simulink model "final_heart_sym3_3_Level_fixed"  (R2021a)
settings: Solver=FixedStepDiscrete  StartTime=0.0  StopTime=8  RelTol=1e-3
undefined symbols (not defined in the file): lambda2
(part 1 of 2)
settings Model: DataTypeOverride=Off  FPTShortcutValueString='{{},{''BaselineRun'',1,1,1,''BaselineRun'','''',{},''M'','''',''''}}'  Creator=Ruth Matienzo  LastModifiedBy=Acer
settings OptimizationCC: BlockReduction=off  ConditionallyExecuteInputs=off  DefaultParameterBehavior=Inlined
settings DebuggingCC: SignalRangeChecking=warning  AlgebraicLoopMsg=error  SingleTaskRateTransMsg=error
settings HardwareCC: ProdBitPerPointer=32  ProdBitPerSizeT=32  ProdBitPerPtrDiffT=32  ProdLargestAtomicFloat=None  ProdIntDivRoundTo=Undefined  ProdEndianess=Unspecified  ProdWordSize=32  ProdHWDeviceType=ASIC/FPGA->ASIC/FPGA  TargetBitPerPointer=64  TargetBitPerSizeT=64  TargetBitPerPtrDiffT=64  TargetLongLongMode=on  TargetIntDivRoundTo=Zero  TargetEndianess=LittleEndian  TargetWordSize=64  TargetHWDeviceType=Custom Processor->MATLAB Host Computer  ProdEqTarget=off

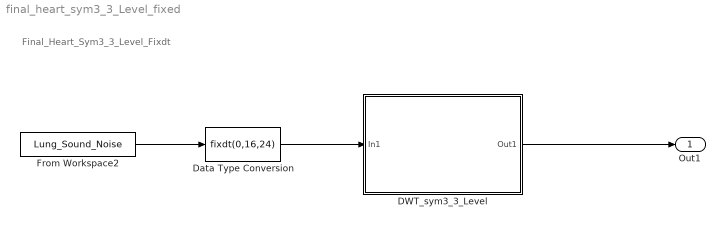
== system final_heart_sym3_3_Level_fixed ==
  note: Final_Heart_Sym3_3_Level_Fixdt
  DWT_sym3_3_Level : Subsystem
  Data Type Conversion : DataTypeConversion  OutDataTypeStr=fixdt(0,16,24)
  From Workspace2 : FromWorkspace  VariableName=Lung_Sound_Noise  OutDataTypeStr=double  SampleTime=1/44100
  Out1 : Outport  OutDataTypeStr=fixdt(1,16,23)  SampleTime=1/44100
  wires:
  Data Type Conversion/1 -> DWT_sym3_3_Level/1(In1)
  DWT_sym3_3_Level/1(Out1) -> Out1/1
  From Workspace2/1 -> Data Type Conversion/1

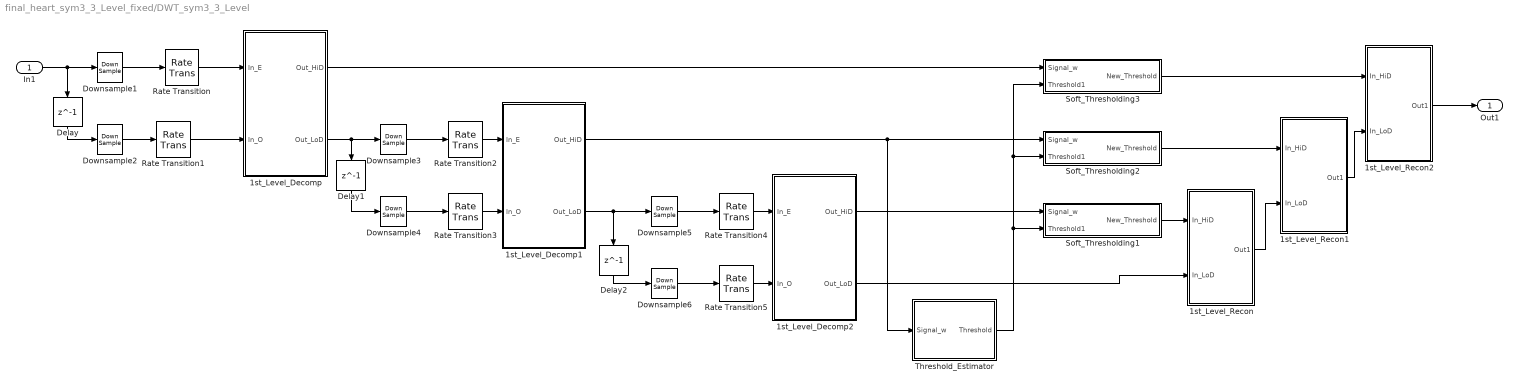
== system final_heart_sym3_3_Level_fixed/DWT_sym3_3_Level ==
  In1 : Inport  OutDataTypeStr=fixdt(0,16,24)
  1st_Level_Decomp : Subsystem
  1st_Level_Decomp1 : Subsystem
  1st_Level_Decomp2 : Subsystem
  1st_Level_Recon : Subsystem
  1st_Level_Recon1 : Subsystem
  1st_Level_Recon2 : Subsystem
  Delay : Delay  DelayLength=1  SampleTime=1/44100
  Delay1 : Delay  DelayLength=1  SampleTime=1/44100
  Delay2 : Delay  DelayLength=1  SampleTime=1/44100
  Downsample{1..6} (6 alike) : DownSample  N=30  RateOptions=Allow multirate processing
  Rate Transition{,1..5} (6 alike) : RateTransition
  Soft_Thresholding1 : Subsystem
  Soft_Thresholding2 : Subsystem
  Soft_Thresholding3 : Subsystem
  Threshold_Estimator : Subsystem
  Out1 : Outport  OutDataTypeStr=fixdt(1,16,23)  SampleTime=1/44100
  wires:
  In1/1 -> Delay/1, Downsample1/1
  Delay1/1 -> Downsample4/1
  1st_Level_Decomp/2(Out_LoD) -> Downsample3/1, Delay1/1
  1st_Level_Recon1/1(Out1) -> 1st_Level_Recon2/2(In_LoD)
  Downsample5/1 -> Rate Transition4/1
  Rate Transition1/1 -> 1st_Level_Decomp/2(In_O)
  Rate Transition/1 -> 1st_Level_Decomp/1(In_E)
  1st_Level_Decomp/1(Out_HiD) -> Soft_Thresholding3/1(Signal_w)
  1st_Level_Decomp1/1(Out_HiD) -> Soft_Thresholding2/1(Signal_w), Threshold_Estimator/1(Signal_w)
  Soft_Thresholding3/1(New_Threshold) -> 1st_Level_Recon2/1(In_HiD)
  1st_Level_Recon/1(Out1) -> 1st_Level_Recon1/2(In_LoD)
  Downsample3/1 -> Rate Transition2/1
  Soft_Thresholding2/1(New_Threshold) -> 1st_Level_Recon1/1(In_HiD)
  Downsample2/1 -> Rate Transition1/1
  Rate Transition5/1 -> 1st_Level_Decomp2/2(In_O)
  Rate Transition2/1 -> 1st_Level_Decomp1/1(In_E)
  Threshold_Estimator/1(Threshold) -> Soft_Thresholding1/2(Threshold1), Soft_Thresholding3/2(Threshold1), Soft_Thresholding2/2(Threshold1)
  Soft_Thresholding1/1(New_Threshold) -> 1st_Level_Recon/1(In_HiD)
  Downsample1/1 -> Rate Transition/1
  1st_Level_Decomp2/2(Out_LoD) -> 1st_Level_Recon/2(In_LoD)
  1st_Level_Decomp2/1(Out_HiD) -> Soft_Thresholding1/1(Signal_w)
  1st_Level_Recon2/1(Out1) -> Out1/1
  Downsample6/1 -> Rate Transition5/1
  Delay/1 -> Downsample2/1
  Rate Transition4/1 -> 1st_Level_Decomp2/1(In_E)
  Rate Transition3/1 -> 1st_Level_Decomp1/2(In_O)
  1st_Level_Decomp1/2(Out_LoD) -> Downsample5/1, Delay2/1
  Delay2/1 -> Downsample6/1
  Downsample4/1 -> Rate Transition3/1

== system final_heart_sym3_3_Level_fixed/DWT_sym3_3_Level/1st_Level_Decomp ==
  In_E : Inport  OutDataTypeStr=fixdt(0,16,24)  SampleTime=1/44100
  In_O : Inport  Port=2  OutDataTypeStr=fixdt(0,16,24)  SampleTime=1/44100
  Add : Sum  AccumDataTypeStr=fixdt(1,16,23)  OutDataTypeStr=fixdt(1,16,24)
  Add1 : Sum  AccumDataTypeStr=fixdt(1,16,22)  OutDataTypeStr=fixdt(1,16,22)
  Delay1 : Delay  DelayLength=1  SampleTime=1/44100
  Delay2 : Delay  DelayLength=1  SampleTime=1/44100
  Gain : Gain  Gain=1/(0.877989329+0.977128821)  ParamDataTypeStr=fixdt(0,16,16)  OutDataTypeStr=fixdt(1,16,25)
  Gain1 : Gain  Gain=1/(0.877989329+0.977128821)  ParamDataTypeStr=fixdt(0,16,16)  OutDataTypeStr=fixdt(1,16,23)
  HiD_Even : Subsystem
  HiD_Odd : Subsystem
  LoD_Even : Subsystem
  LoD_Odd : Subsystem
  Out_HiD : Outport  OutDataTypeStr=fixdt(1,16,25)  SampleTime=1/44100  VectorParamsAs1DForOutWhenUnconnected=off
  Out_LoD : Outport  Port=2  OutDataTypeStr=fixdt(1,16,23)  SampleTime=1/44100  VectorParamsAs1DForOutWhenUnconnected=off
  wires:
  HiD_Odd/1(Out_HiD_o) -> Add/2
  HiD_Even/1(Out_HiD_e) -> Add/1
  LoD_Odd/1(Out_LoD_o) -> Add1/2
  LoD_Even/1(Out_LoD_e) -> Add1/1
  In_E/1 -> LoD_Even/1(In_LoD_e), HiD_Even/1(In_HiD_e)
  In_O/1 -> LoD_Odd/1(In_LoD_o), HiD_Odd/1(In_HiD_o)
  Gain/1 -> Delay1/1
  Delay1/1 -> Out_HiD/1
  Delay2/1 -> Out_LoD/1
  Add/1 -> Gain/1
  Add1/1 -> Gain1/1
  Gain1/1 -> Delay2/1

== system final_heart_sym3_3_Level_fixed/DWT_sym3_3_Level/1st_Level_Decomp1 ==
  In_E : Inport  OutDataTypeStr=fixdt(1,16,23)  SampleTime=1/44100
  In_O : Inport  Port=2  OutDataTypeStr=fixdt(1,16,23)  SampleTime=1/44100
  Add : Sum  AccumDataTypeStr=fixdt(1,16,24)  OutDataTypeStr=fixdt(1,16,26)
  Add1 : Sum  AccumDataTypeStr=fixdt(1,16,23)  OutDataTypeStr=fixdt(1,16,23)
  Delay1 : Delay  DelayLength=1  SampleTime=1/44100
  Delay2 : Delay  DelayLength=1  SampleTime=1/44100
  Gain : Gain  Gain=1/(0.877989329+0.977128821)  ParamDataTypeStr=fixdt(0,16,16)  OutDataTypeStr=fixdt(1,16,27)
  Gain1 : Gain  Gain=1/(0.877989329+0.977128821)  ParamDataTypeStr=fixdt(0,16,16)  OutDataTypeStr=fixdt(1,16,24)
  HiD_Even : Subsystem
  HiD_Odd : Subsystem
  LoD_Even : Subsystem
  LoD_Odd : Subsystem
  Out_HiD : Outport  OutDataTypeStr=fixdt(1,16,27)  SampleTime=1/44100  VectorParamsAs1DForOutWhenUnconnected=off
  Out_LoD : Outport  Port=2  OutDataTypeStr=fixdt(1,16,24)  SampleTime=1/44100  VectorParamsAs1DForOutWhenUnconnected=off
  wires:
  HiD_Odd/1(Out_HiD_o) -> Add/2
  HiD_Even/1(Out_HiD_e) -> Add/1
  LoD_Odd/1(Out_LoD_o) -> Add1/2
  LoD_Even/1(Out_LoD_e) -> Add1/1
  In_E/1 -> LoD_Even/1(In_LoD_e), HiD_Even/1(In_HiD_e)
  In_O/1 -> LoD_Odd/1(In_LoD_o), HiD_Odd/1(In_HiD_o)
  Gain/1 -> Delay1/1
  Delay1/1 -> Out_HiD/1
  Delay2/1 -> Out_LoD/1
  Add/1 -> Gain/1
  Add1/1 -> Gain1/1
  Gain1/1 -> Delay2/1

== system final_heart_sym3_3_Level_fixed/DWT_sym3_3_Level/1st_Level_Decomp2 ==
  In_E : Inport  OutDataTypeStr=fixdt(1,16,24)  SampleTime=1/44100
  In_O : Inport  Port=2  OutDataTypeStr=fixdt(1,16,24)  SampleTime=1/44100
  Add : Sum  AccumDataTypeStr=fixdt(1,16,24)  OutDataTypeStr=fixdt(1,16,26)
  Add1 : Sum  AccumDataTypeStr=fixdt(1,16,23)  OutDataTypeStr=fixdt(1,16,23)
  Delay1 : Delay  DelayLength=1  SampleTime=1/44100
  Delay2 : Delay  DelayLength=1  SampleTime=1/44100
  Gain : Gain  Gain=1/(0.877989329+0.977128821)  ParamDataTypeStr=fixdt(0,16,16)  OutDataTypeStr=fixdt(1,16,27)
  Gain1 : Gain  Gain=1/(0.877989329+0.977128821)  ParamDataTypeStr=fixdt(0,16,16)  OutDataTypeStr=fixdt(1,16,24)
  HiD_Even : Subsystem
  HiD_Odd : Subsystem
  LoD_Even : Subsystem
  LoD_Odd : Subsystem
  Out_HiD : Outport  OutDataTypeStr=fixdt(1,16,27)  SampleTime=1/44100  VectorParamsAs1DForOutWhenUnconnected=off
  Out_LoD : Outport  Port=2  OutDataTypeStr=fixdt(1,16,24)  SampleTime=1/44100  VectorParamsAs1DForOutWhenUnconnected=off
  wires:
  HiD_Odd/1(Out_HiD_o) -> Add/2
  HiD_Even/1(Out_HiD_e) -> Add/1
  LoD_Odd/1(Out_LoD_o) -> Add1/2
  LoD_Even/1(Out_LoD_e) -> Add1/1
  In_E/1 -> LoD_Even/1(In_LoD_e), HiD_Even/1(In_HiD_e)
  In_O/1 -> LoD_Odd/1(In_LoD_o), HiD_Odd/1(In_HiD_o)
  Gain/1 -> Delay1/1
  Delay1/1 -> Out_HiD/1
  Delay2/1 -> Out_LoD/1
  Add/1 -> Gain/1
  Add1/1 -> Gain1/1
  Gain1/1 -> Delay2/1

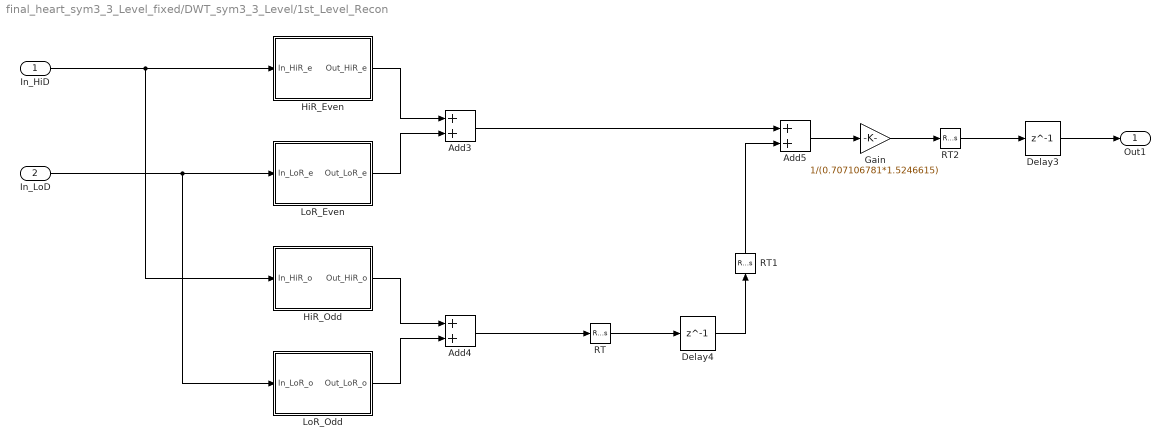
== system final_heart_sym3_3_Level_fixed/DWT_sym3_3_Level/1st_Level_Recon ==
  In_HiD : Inport  OutDataTypeStr=fixdt(1,16,28)  SampleTime=1/44100
  In_LoD : Inport  Port=2  OutDataTypeStr=fixdt(1,16,24)  SampleTime=1/44100
  Add3 : Sum  AccumDataTypeStr=fixdt(1,16,24)  OutDataTypeStr=fixdt(1,16,24)
  Add4 : Sum  AccumDataTypeStr=fixdt(1,16,24)  OutDataTypeStr=fixdt(1,16,24)
  Add5 : Sum  AccumDataTypeStr=fixdt(1,16,23)  OutDataTypeStr=fixdt(1,16,23)
  Delay3 : Delay  DelayLength=1  SampleTime=1/44100
  Delay4 : Delay  DelayLength=1  SampleTime=1/44100
  Gain : Gain  Gain=1/(0.707106781*1.5246615)  ParamDataTypeStr=fixdt(0,16,16)  OutDataTypeStr=fixdt(1,16,24)
  HiR_Even : Subsystem
  HiR_Odd : Subsystem
  LoR_Even : Subsystem
  LoR_Odd : Subsystem
  RT : RateTransition
  RT1 : RateTransition
  RT2 : RateTransition
  Out1 : Outport  OutDataTypeStr=fixdt(1,16,24)  SampleTime=1/44100
  wires:
  In_HiD/1 -> HiR_Odd/1(In_HiR_o), HiR_Even/1(In_HiR_e)
  HiR_Even/1(Out_HiR_e) -> Add3/1
  In_LoD/1 -> LoR_Odd/1(In_LoR_o), LoR_Even/1(In_LoR_e)
  LoR_Even/1(Out_LoR_e) -> Add3/2
  HiR_Odd/1(Out_HiR_o) -> Add4/1
  LoR_Odd/1(Out_LoR_o) -> Add4/2
  RT/1 -> Delay4/1
  Delay3/1 -> Out1/1
  RT1/1 -> Add5/2
  RT2/1 -> Delay3/1
  Delay4/1 -> RT1/1
  Add5/1 -> Gain/1
  Gain/1 -> RT2/1
  Add3/1 -> Add5/1
  Add4/1 -> RT/1

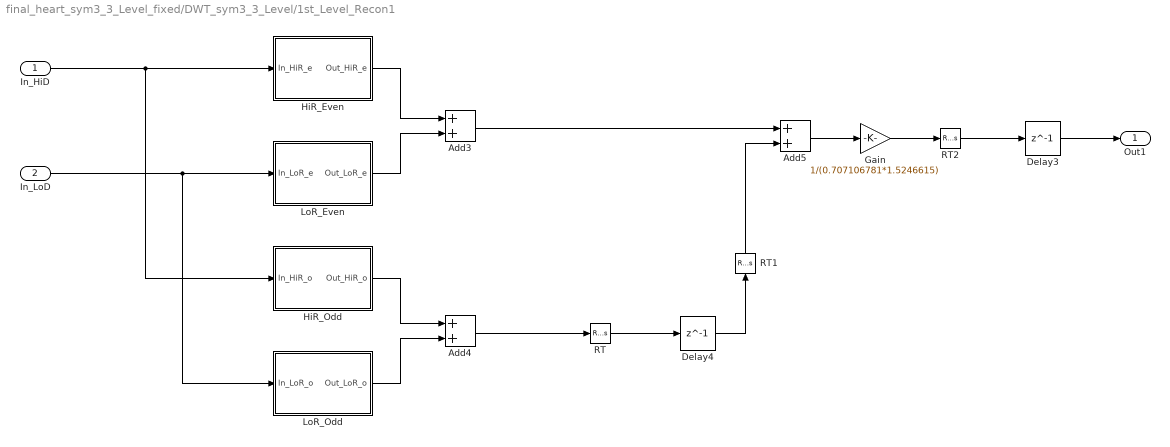
== system final_heart_sym3_3_Level_fixed/DWT_sym3_3_Level/1st_Level_Recon1 ==
  In_HiD : Inport  OutDataTypeStr=fixdt(1,16,28)  SampleTime=1/44100
  In_LoD : Inport  Port=2  OutDataTypeStr=fixdt(1,16,24)  SampleTime=1/44100
  Add3 : Sum  AccumDataTypeStr=fixdt(1,16,24)  OutDataTypeStr=fixdt(1,16,24)
  Add4 : Sum  AccumDataTypeStr=fixdt(1,16,24)  OutDataTypeStr=fixdt(1,16,24)
  Add5 : Sum  AccumDataTypeStr=fixdt(1,16,23)  OutDataTypeStr=fixdt(1,16,23)
  Delay3 : Delay  DelayLength=1  SampleTime=1/44100
  Delay4 : Delay  DelayLength=1  SampleTime=1/44100
  Gain : Gain  Gain=1/(0.707106781*1.5246615)  ParamDataTypeStr=fixdt(0,16,16)  OutDataTypeStr=fixdt(1,16,23)
  HiR_Even : Subsystem
  HiR_Odd : Subsystem
  LoR_Even : Subsystem
  LoR_Odd : Subsystem
  RT : RateTransition
  RT1 : RateTransition
  RT2 : RateTransition
  Out1 : Outport  OutDataTypeStr=fixdt(1,16,23)  SampleTime=1/44100
  wires:
  In_HiD/1 -> HiR_Odd/1(In_HiR_o), HiR_Even/1(In_HiR_e)
  HiR_Even/1(Out_HiR_e) -> Add3/1
  In_LoD/1 -> LoR_Odd/1(In_LoR_o), LoR_Even/1(In_LoR_e)
  LoR_Even/1(Out_LoR_e) -> Add3/2
  HiR_Odd/1(Out_HiR_o) -> Add4/1
  LoR_Odd/1(Out_LoR_o) -> Add4/2
  RT/1 -> Delay4/1
  Delay3/1 -> Out1/1
  RT1/1 -> Add5/2
  RT2/1 -> Delay3/1
  Delay4/1 -> RT1/1
  Add5/1 -> Gain/1
  Gain/1 -> RT2/1
  Add3/1 -> Add5/1
  Add4/1 -> RT/1

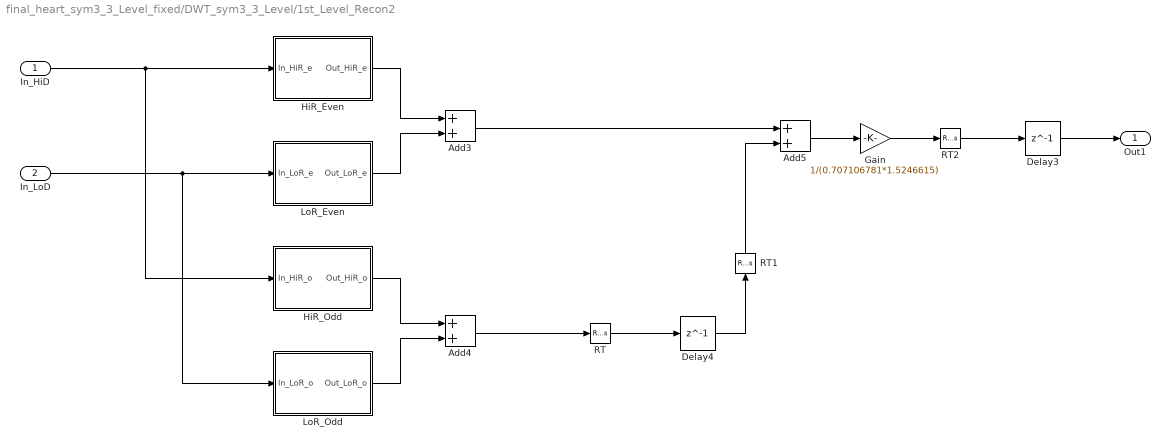
== system final_heart_sym3_3_Level_fixed/DWT_sym3_3_Level/1st_Level_Recon2 ==
  In_HiD : Inport  OutDataTypeStr=fixdt(1,16,28)  SampleTime=1/44100
  In_LoD : Inport  Port=2  OutDataTypeStr=fixdt(1,16,23)  SampleTime=1/44100
  Add3 : Sum  AccumDataTypeStr=fixdt(1,16,24)  OutDataTypeStr=fixdt(1,16,24)
  Add4 : Sum  AccumDataTypeStr=fixdt(1,16,24)  OutDataTypeStr=fixdt(1,16,24)
  Add5 : Sum  AccumDataTypeStr=fixdt(1,16,23)  OutDataTypeStr=fixdt(1,16,23)
  Delay3 : Delay  DelayLength=1  SampleTime=1/44100
  Delay4 : Delay  DelayLength=1  SampleTime=1/44100
  Gain : Gain  Gain=1/(0.707106781*1.5246615)  ParamDataTypeStr=fixdt(0,16,16)  OutDataTypeStr=fixdt(1,16,23)
  HiR_Even : Subsystem
  HiR_Odd : Subsystem
  LoR_Even : Subsystem
  LoR_Odd : Subsystem
  RT : RateTransition
  RT1 : RateTransition
  RT2 : RateTransition
  Out1 : Outport  OutDataTypeStr=fixdt(1,16,23)  SampleTime=1/44100
  wires:
  In_HiD/1 -> HiR_Odd/1(In_HiR_o), HiR_Even/1(In_HiR_e)
  HiR_Even/1(Out_HiR_e) -> Add3/1
  In_LoD/1 -> LoR_Odd/1(In_LoR_o), LoR_Even/1(In_LoR_e)
  LoR_Even/1(Out_LoR_e) -> Add3/2
  HiR_Odd/1(Out_HiR_o) -> Add4/1
  LoR_Odd/1(Out_LoR_o) -> Add4/2
  RT/1 -> Delay4/1
  Delay3/1 -> Out1/1
  RT1/1 -> Add5/2
  RT2/1 -> Delay3/1
  Delay4/1 -> RT1/1
  Add5/1 -> Gain/1
  Gain/1 -> RT2/1
  Add3/1 -> Add5/1
  Add4/1 -> RT/1

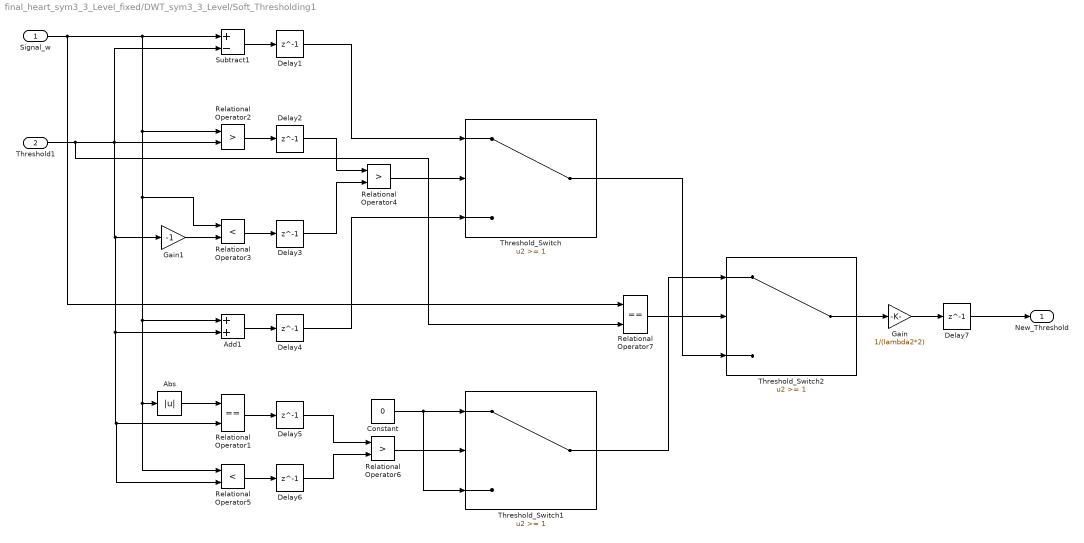
== system final_heart_sym3_3_Level_fixed/DWT_sym3_3_Level/Soft_Thresholding1 ==
  Signal_w : Inport  OutDataTypeStr=fixdt(1,16,27)  SampleTime=1/44100
  Threshold1 : Inport  Port=2  OutDataTypeStr=fixdt(0,16,26)  SampleTime=1/44100
  Abs : Abs  OutDataTypeStr=fixdt(0,16,28)
  Add1 : Sum  AccumDataTypeStr=fixdt(1,16,25)  OutDataTypeStr=fixdt(1,16,25)
  Constant : Constant  Value=0  OutDataTypeStr=fixdt(1,16,4)  SampleTime=1/44100
  Delay{1..7} (7 alike) : Delay  DelayLength=1  SampleTime=1/44100
  Gain : Gain  Gain=1/(lambda2*2)  ParamDataTypeStr=fixdt(0,16,19)  OutDataTypeStr=fixdt(1,16,28)
  Gain1 : Gain  Gain=-1  ParamDataTypeStr=fixdt(1,16,15)  OutMin=-1  OutMax=-0.99  OutDataTypeStr=fixdt(1,16,15)
  Relational Operator1 : RelationalOperator  Operator===  OutDataTypeStr=boolean  RndMeth=Simplest
  Relational Operator2 : RelationalOperator  Operator=>  OutDataTypeStr=boolean  RndMeth=Simplest
  Relational Operator3 : RelationalOperator  Operator=<  OutDataTypeStr=boolean  RndMeth=Simplest
  Relational Operator4 : RelationalOperator  Operator=>  OutDataTypeStr=boolean  RndMeth=Simplest
  Relational Operator5 : RelationalOperator  Operator=<  OutDataTypeStr=boolean  RndMeth=Simplest
  Relational Operator6 : RelationalOperator  Operator=>  OutDataTypeStr=boolean  RndMeth=Simplest
  Relational Operator7 : RelationalOperator  Operator===  OutDataTypeStr=boolean  RndMeth=Simplest
  Subtract1 : Sum  Inputs=+-  AccumDataTypeStr=fixdt(1,16,25)  OutDataTypeStr=fixdt(1,16,25)
  Threshold_Switch : Switch  Threshold=1  OutDataTypeStr=fixdt(1,16,25)
  Threshold_Switch1 : Switch  Threshold=1  OutDataTypeStr=fixdt(1,16,4)
  Threshold_Switch2 : Switch  Threshold=1  OutDataTypeStr=fixdt(1,16,25)
  New_Threshold : Outport  OutDataTypeStr=fixdt(1,16,28)  SampleTime=1/44100
  wires:
  Threshold_Switch/1 -> Threshold_Switch2/3
  Relational Operator6/1 -> Threshold_Switch1/2
  Gain1/1 -> Relational Operator3/2
  Delay4/1 -> Threshold_Switch/3
  Add1/1 -> Delay4/1
  Delay2/1 -> Relational Operator4/1
  Delay3/1 -> Relational Operator4/2
  Delay1/1 -> Threshold_Switch/1
  Relational Operator2/1 -> Delay2/1
  Relational Operator3/1 -> Delay3/1
  Relational Operator5/1 -> Delay6/1
  Delay6/1 -> Relational Operator6/2
  Delay5/1 -> Relational Operator6/1
  Threshold1/1 -> Relational Operator2/2, Subtract1/2, Relational Operator5/2, Relational Operator1/2, Add1/2, Gain1/1, Relational Operator7/2
  Abs/1 -> Relational Operator1/1
  Relational Operator4/1 -> Threshold_Switch/2
  Subtract1/1 -> Delay1/1
  Constant/1 -> Threshold_Switch1/3, Threshold_Switch1/1
  Signal_w/1 -> Subtract1/1, Relational Operator2/1, Relational Operator5/1, Abs/1, Add1/1, Relational Operator3/1, Relational Operator7/1
  Relational Operator7/1 -> Threshold_Switch2/2
  Relational Operator1/1 -> Delay5/1
  Threshold_Switch1/1 -> Threshold_Switch2/1
  Delay7/1 -> New_Threshold/1
  Threshold_Switch2/1 -> Gain/1
  Gain/1 -> Delay7/1

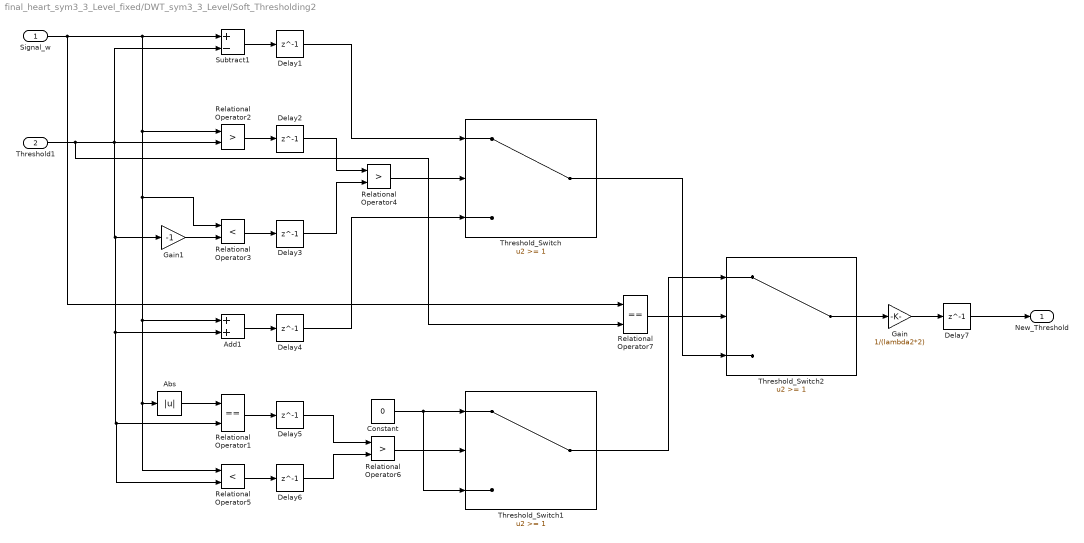
== system final_heart_sym3_3_Level_fixed/DWT_sym3_3_Level/Soft_Thresholding2 ==
  Signal_w : Inport  OutDataTypeStr=fixdt(1,16,27)  SampleTime=1/44100
  Threshold1 : Inport  Port=2  OutDataTypeStr=fixdt(0,16,26)  SampleTime=1/44100
  Abs : Abs  OutDataTypeStr=fixdt(0,16,28)
  Add1 : Sum  AccumDataTypeStr=fixdt(1,16,25)  OutDataTypeStr=fixdt(1,16,25)
  Constant : Constant  Value=0  OutDataTypeStr=fixdt(1,16,4)  SampleTime=1/44100
  Delay{1..7} (7 alike) : Delay  DelayLength=1  SampleTime=1/44100
  Gain : Gain  Gain=1/(lambda2*2)  ParamDataTypeStr=fixdt(0,16,19)  OutDataTypeStr=fixdt(1,16,28)
  Gain1 : Gain  Gain=-1  ParamDataTypeStr=fixdt(1,16,15)  OutMin=-1  OutMax=-0.99  OutDataTypeStr=fixdt(1,16,15)
  Relational Operator1 : RelationalOperator  Operator===  OutDataTypeStr=boolean  RndMeth=Simplest
  Relational Operator2 : RelationalOperator  Operator=>  OutDataTypeStr=boolean  RndMeth=Simplest
  Relational Operator3 : RelationalOperator  Operator=<  OutDataTypeStr=boolean  RndMeth=Simplest
  Relational Operator4 : RelationalOperator  Operator=>  OutDataTypeStr=boolean  RndMeth=Simplest
  Relational Operator5 : RelationalOperator  Operator=<  OutDataTypeStr=boolean  RndMeth=Simplest
  Relational Operator6 : RelationalOperator  Operator=>  OutDataTypeStr=boolean  RndMeth=Simplest
  Relational Operator7 : RelationalOperator  Operator===  OutDataTypeStr=boolean  RndMeth=Simplest
  Subtract1 : Sum  Inputs=+-  AccumDataTypeStr=fixdt(1,16,25)  OutDataTypeStr=fixdt(1,16,25)
  Threshold_Switch : Switch  Threshold=1  OutDataTypeStr=fixdt(1,16,25)
  Threshold_Switch1 : Switch  Threshold=1  OutDataTypeStr=fixdt(1,16,4)
  Threshold_Switch2 : Switch  Threshold=1  OutDataTypeStr=fixdt(1,16,25)
  New_Threshold : Outport  OutDataTypeStr=fixdt(1,16,28)  SampleTime=1/44100
  wires:
  Threshold_Switch/1 -> Threshold_Switch2/3
  Relational Operator6/1 -> Threshold_Switch1/2
  Gain1/1 -> Relational Operator3/2
  Delay4/1 -> Threshold_Switch/3
  Add1/1 -> Delay4/1
  Delay2/1 -> Relational Operator4/1
  Delay3/1 -> Relational Operator4/2
  Delay1/1 -> Threshold_Switch/1
  Relational Operator2/1 -> Delay2/1
  Relational Operator3/1 -> Delay3/1
  Relational Operator5/1 -> Delay6/1
  Delay6/1 -> Relational Operator6/2
  Delay5/1 -> Relational Operator6/1
  Threshold1/1 -> Relational Operator2/2, Subtract1/2, Relational Operator5/2, Relational Operator1/2, Add1/2, Gain1/1, Relational Operator7/2
  Abs/1 -> Relational Operator1/1
  Relational Operator4/1 -> Threshold_Switch/2
  Subtract1/1 -> Delay1/1
  Constant/1 -> Threshold_Switch1/3, Threshold_Switch1/1
  Signal_w/1 -> Subtract1/1, Relational Operator2/1, Relational Operator5/1, Abs/1, Add1/1, Relational Operator3/1, Relational Operator7/1
  Relational Operator7/1 -> Threshold_Switch2/2
  Relational Operator1/1 -> Delay5/1
  Threshold_Switch1/1 -> Threshold_Switch2/1
  Delay7/1 -> New_Threshold/1
  Threshold_Switch2/1 -> Gain/1
  Gain/1 -> Delay7/1

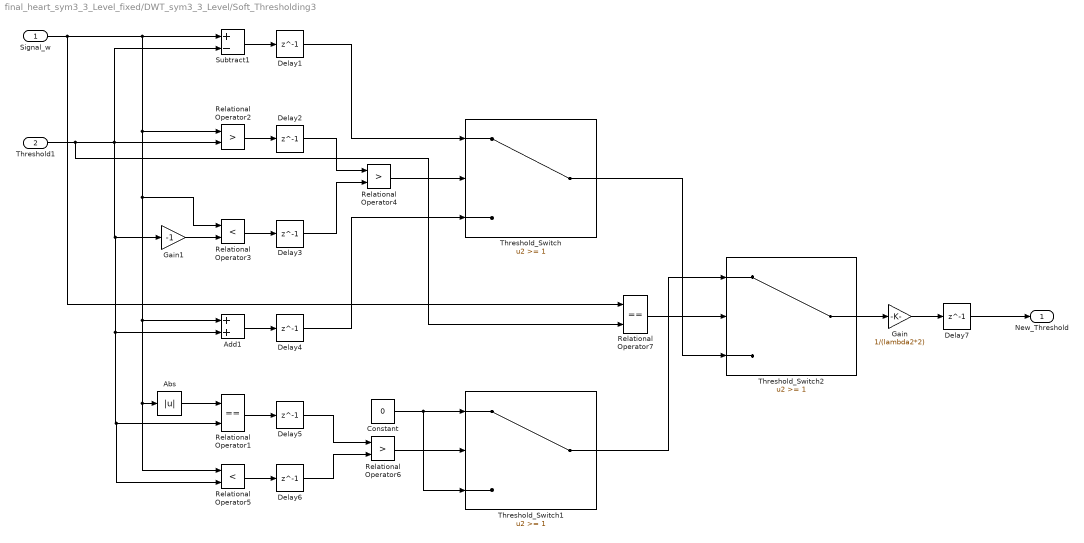
== system final_heart_sym3_3_Level_fixed/DWT_sym3_3_Level/Soft_Thresholding3 ==
  Signal_w : Inport  OutDataTypeStr=fixdt(1,16,25)  SampleTime=1/44100
  Threshold1 : Inport  Port=2  OutDataTypeStr=fixdt(0,16,26)  SampleTime=1/44100
  Abs : Abs  OutDataTypeStr=fixdt(0,16,26)
  Add1 : Sum  AccumDataTypeStr=fixdt(1,16,25)  OutDataTypeStr=fixdt(1,16,25)
  Constant : Constant  Value=0  OutDataTypeStr=fixdt(1,16,4)  SampleTime=1/44100
  Delay{1..7} (7 alike) : Delay  DelayLength=1  SampleTime=1/44100
  Gain : Gain  Gain=1/(lambda2*2)  ParamDataTypeStr=fixdt(0,16,19)  OutDataTypeStr=fixdt(1,16,28)
  Gain1 : Gain  Gain=-1  ParamDataTypeStr=fixdt(1,16,15)  OutMin=-1  OutMax=-0.99  OutDataTypeStr=fixdt(1,16,15)
  Relational Operator1 : RelationalOperator  Operator===  OutDataTypeStr=boolean  RndMeth=Simplest
  Relational Operator2 : RelationalOperator  Operator=>  OutDataTypeStr=boolean  RndMeth=Simplest
  Relational Operator3 : RelationalOperator  Operator=<  OutDataTypeStr=boolean  RndMeth=Simplest
  Relational Operator4 : RelationalOperator  Operator=>  OutDataTypeStr=boolean  RndMeth=Simplest
  Relational Operator5 : RelationalOperator  Operator=<  OutDataTypeStr=boolean  RndMeth=Simplest
  Relational Operator6 : RelationalOperator  Operator=>  OutDataTypeStr=boolean  RndMeth=Simplest
  Relational Operator7 : RelationalOperator  Operator===  OutDataTypeStr=boolean  RndMeth=Simplest
  Subtract1 : Sum  Inputs=+-  AccumDataTypeStr=fixdt(1,16,25)  OutDataTypeStr=fixdt(1,16,25)
  Threshold_Switch : Switch  Threshold=1  OutDataTypeStr=fixdt(1,16,25)
  Threshold_Switch1 : Switch  Threshold=1  OutDataTypeStr=fixdt(1,16,4)
  Threshold_Switch2 : Switch  Threshold=1  OutDataTypeStr=fixdt(1,16,25)
  New_Threshold : Outport  OutDataTypeStr=fixdt(1,16,28)  SampleTime=1/44100
  wires:
  Threshold_Switch/1 -> Threshold_Switch2/3
  Relational Operator6/1 -> Threshold_Switch1/2
  Gain1/1 -> Relational Operator3/2
  Delay4/1 -> Threshold_Switch/3
  Add1/1 -> Delay4/1
  Delay2/1 -> Relational Operator4/1
  Delay3/1 -> Relational Operator4/2
  Delay1/1 -> Threshold_Switch/1
  Relational Operator2/1 -> Delay2/1
  Relational Operator3/1 -> Delay3/1
  Relational Operator5/1 -> Delay6/1
  Delay6/1 -> Relational Operator6/2
  Delay5/1 -> Relational Operator6/1
  Threshold1/1 -> Relational Operator2/2, Subtract1/2, Relational Operator5/2, Relational Operator1/2, Add1/2, Gain1/1, Relational Operator7/2
  Abs/1 -> Relational Operator1/1
  Relational Operator4/1 -> Threshold_Switch/2
  Subtract1/1 -> Delay1/1
  Constant/1 -> Threshold_Switch1/3, Threshold_Switch1/1
  Signal_w/1 -> Subtract1/1, Relational Operator2/1, Relational Operator5/1, Abs/1, Add1/1, Relational Operator3/1, Relational Operator7/1
  Relational Operator7/1 -> Threshold_Switch2/2
  Relational Operator1/1 -> Delay5/1
  Threshold_Switch1/1 -> Threshold_Switch2/1
  Delay7/1 -> New_Threshold/1
  Threshold_Switch2/1 -> Gain/1
  Gain/1 -> Delay7/1

== system final_heart_sym3_3_Level_fixed/DWT_sym3_3_Level/Threshold_Estimator ==
  Signal_w : Inport  OutDataTypeStr=fixdt(1,16,27)  SampleTime=1/44100
  Absolute_Value1 : Subsystem
  Length : Constant  Value=lambda2  OutDataTypeStr=fixdt(0,16,13)  SampleTime=1/44100
  Median2 : Subsystem
  Multiply : Product  OutDataTypeStr=fixdt(0,16,26)
  Threshold : Outport  OutDataTypeStr=fixdt(0,16,26)  SampleTime=1/44100  VectorParamsAs1DForOutWhenUnconnected=off
  wires:
  Length/1 -> Multiply/2
  Median2/1(Median) -> Multiply/1
  Absolute_Value1/1(Out_Abs) -> Median2/1(Signal_w3)
  Signal_w/1 -> Absolute_Value1/1(Signal_w4)
  Multiply/1 -> Threshold/1

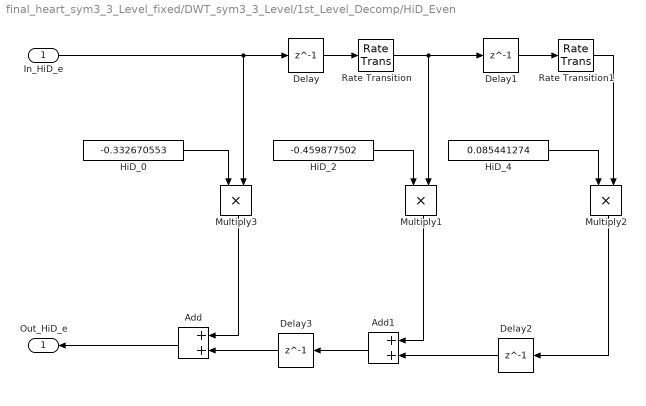
== system final_heart_sym3_3_Level_fixed/DWT_sym3_3_Level/1st_Level_Decomp/HiD_Even ==
  In_HiD_e : Inport  OutDataTypeStr=fixdt(0,16,24)  SampleTime=1/44100
  Add : Sum  AccumDataTypeStr=fixdt(1,16,23)  OutDataTypeStr=fixdt(1,16,23)
  Add1 : Sum  AccumDataTypeStr=fixdt(1,16,24)  OutDataTypeStr=fixdt(1,16,24)
  Delay{,1..3} (4 alike) : Delay  DelayLength=1  SampleTime=1/44100
  HiD_0 : Constant  Value=-0.332670553  OutDataTypeStr=fixdt(1,16,16)  SampleTime=1/44100
  HiD_2 : Constant  Value=-0.459877502  OutDataTypeStr=fixdt(1,16,16)  SampleTime=1/44100
  HiD_4 : Constant  Value=0.085441274  OutDataTypeStr=fixdt(0,16,19)  SampleTime=1/44100
  Multiply1 : Product  OutDataTypeStr=fixdt(1,16,15)
  Multiply2 : Product  OutDataTypeStr=fixdt(0,16,27)
  Multiply3 : Product  OutDataTypeStr=fixdt(1,16,15)
  Rate Transition : RateTransition
  Rate Transition1 : RateTransition
  Out_HiD_e : Outport  OutDataTypeStr=fixdt(1,16,23)  SampleTime=1/44100  VectorParamsAs1DForOutWhenUnconnected=off
  wires:
  In_HiD_e/1 -> Multiply3/2, Delay/1
  Multiply3/1 -> Add/1
  HiD_0/1 -> Multiply3/1
  HiD_2/1 -> Multiply1/1
  Add/1 -> Out_HiD_e/1
  Multiply2/1 -> Delay2/1
  Multiply1/1 -> Add1/1
  Delay2/1 -> Add1/2
  Add1/1 -> Delay3/1
  Delay3/1 -> Add/2
  HiD_4/1 -> Multiply2/1
  Rate Transition1/1 -> Multiply2/2
  Delay1/1 -> Rate Transition1/1
  Rate Transition/1 -> Multiply1/2, Delay1/1
  Delay/1 -> Rate Transition/1

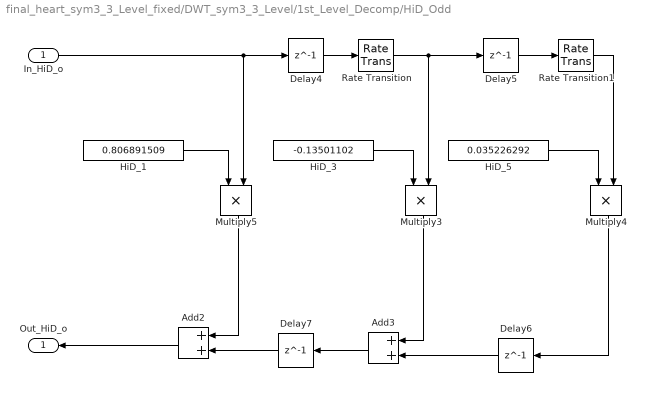
== system final_heart_sym3_3_Level_fixed/DWT_sym3_3_Level/1st_Level_Decomp/HiD_Odd ==
  In_HiD_o : Inport  OutDataTypeStr=fixdt(0,16,24)  SampleTime=1/44100
  Add2 : Sum  AccumDataTypeStr=fixdt(1,16,23)  OutDataTypeStr=fixdt(1,16,23)
  Add3 : Sum  AccumDataTypeStr=fixdt(1,16,26)  OutDataTypeStr=fixdt(1,16,26)
  Delay{4..7} (4 alike) : Delay  DelayLength=1  SampleTime=1/44100
  HiD_1 : Constant  Value=0.806891509  OutDataTypeStr=fixdt(0,16,16)  SampleTime=1/44100
  HiD_3 : Constant  Value=-0.13501102  OutDataTypeStr=fixdt(1,16,17)  SampleTime=1/44100
  HiD_5 : Constant  Value=0.035226292  OutDataTypeStr=fixdt(0,16,20)  SampleTime=1/44100
  Multiply3 : Product  OutDataTypeStr=fixdt(1,16,15)
  Multiply4 : Product  OutDataTypeStr=fixdt(0,16,29)
  Multiply5 : Product  OutDataTypeStr=fixdt(0,16,24)
  Rate Transition : RateTransition
  Rate Transition1 : RateTransition
  Out_HiD_o : Outport  OutDataTypeStr=fixdt(1,16,23)  SampleTime=1/44100  VectorParamsAs1DForOutWhenUnconnected=off
  wires:
  Delay5/1 -> Rate Transition1/1
  Rate Transition1/1 -> Multiply4/2
  HiD_3/1 -> Multiply3/1
  Add3/1 -> Delay7/1
  Delay7/1 -> Add2/2
  HiD_5/1 -> Multiply4/1
  In_HiD_o/1 -> Multiply5/2, Delay4/1
  Multiply5/1 -> Add2/1
  Add2/1 -> Out_HiD_o/1
  Multiply4/1 -> Delay6/1
  Multiply3/1 -> Add3/1
  Delay4/1 -> Rate Transition/1
  HiD_1/1 -> Multiply5/1
  Delay6/1 -> Add3/2
  Rate Transition/1 -> Multiply3/2, Delay5/1

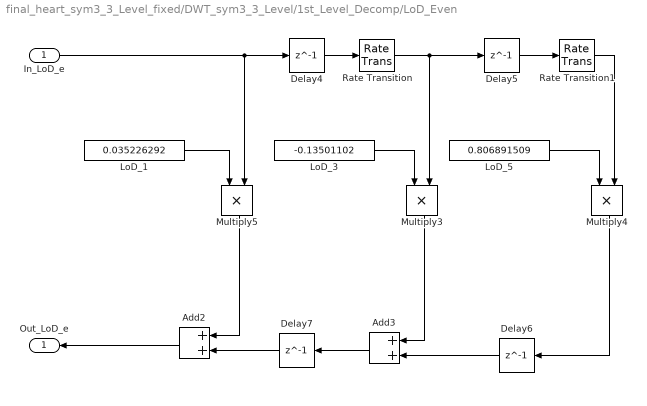
== system final_heart_sym3_3_Level_fixed/DWT_sym3_3_Level/1st_Level_Decomp/LoD_Even ==
  In_LoD_e : Inport  OutDataTypeStr=fixdt(0,16,24)  SampleTime=1/44100
  Add2 : Sum  AccumDataTypeStr=fixdt(1,16,23)  OutDataTypeStr=fixdt(1,16,23)
  Add3 : Sum  AccumDataTypeStr=fixdt(1,16,23)  OutDataTypeStr=fixdt(1,16,23)
  Delay{4..7} (4 alike) : Delay  DelayLength=1  SampleTime=1/44100
  LoD_1 : Constant  Value=0.035226292  OutDataTypeStr=fixdt(0,16,20)  SampleTime=1/44100
  LoD_3 : Constant  Value=-0.13501102  OutDataTypeStr=fixdt(1,16,17)  SampleTime=1/44100
  LoD_5 : Constant  Value=0.806891509  OutDataTypeStr=fixdt(0,16,16)  SampleTime=1/44100
  Multiply3 : Product  OutDataTypeStr=fixdt(1,16,15)
  Multiply4 : Product  OutDataTypeStr=fixdt(0,16,24)
  Multiply5 : Product  OutDataTypeStr=fixdt(0,16,29)
  Rate Transition : RateTransition
  Rate Transition1 : RateTransition
  Out_LoD_e : Outport  OutDataTypeStr=fixdt(1,16,23)  SampleTime=1/44100  VectorParamsAs1DForOutWhenUnconnected=off
  wires:
  Delay5/1 -> Rate Transition1/1
  Rate Transition1/1 -> Multiply4/2
  LoD_3/1 -> Multiply3/1
  Add3/1 -> Delay7/1
  Delay7/1 -> Add2/2
  LoD_5/1 -> Multiply4/1
  In_LoD_e/1 -> Multiply5/2, Delay4/1
  Multiply5/1 -> Add2/1
  Add2/1 -> Out_LoD_e/1
  Multiply4/1 -> Delay6/1
  Multiply3/1 -> Add3/1
  Delay4/1 -> Rate Transition/1
  LoD_1/1 -> Multiply5/1
  Delay6/1 -> Add3/2
  Rate Transition/1 -> Multiply3/2, Delay5/1

== system final_heart_sym3_3_Level_fixed/DWT_sym3_3_Level/1st_Level_Decomp/LoD_Odd ==
  In_LoD_o : Inport  OutDataTypeStr=fixdt(0,16,24)  SampleTime=1/44100
  Add2 : Sum  AccumDataTypeStr=fixdt(1,16,23)  OutDataTypeStr=fixdt(1,16,23)
  Add3 : Sum  AccumDataTypeStr=fixdt(0,16,24)  OutDataTypeStr=fixdt(0,16,24)
  Delay{4..7} (4 alike) : Delay  DelayLength=1  SampleTime=1/44100
  LoD_1 : Constant  Value=-0.085441274  OutDataTypeStr=fixdt(1,16,18)  SampleTime=1/44100
  LoD_3 : Constant  Value=0.459877502  OutDataTypeStr=fixdt(0,16,17)  SampleTime=1/44100
  LoD_5 : Constant  Value=0.332670553  OutDataTypeStr=fixdt(0,16,17)  SampleTime=1/44100
  Multiply3 : Product  OutDataTypeStr=fixdt(0,16,25)
  Multiply4 : Product  OutDataTypeStr=fixdt(0,16,25)
  Multiply5 : Product  OutDataTypeStr=fixdt(1,16,15)
  Rate Transition : RateTransition
  Rate Transition1 : RateTransition
  Out_LoD_o : Outport  OutDataTypeStr=fixdt(1,16,23)  SampleTime=1/44100  VectorParamsAs1DForOutWhenUnconnected=off
  wires:
  Delay5/1 -> Rate Transition1/1
  Rate Transition1/1 -> Multiply4/2
  LoD_3/1 -> Multiply3/1
  Add3/1 -> Delay7/1
  Delay7/1 -> Add2/2
  LoD_5/1 -> Multiply4/1
  In_LoD_o/1 -> Multiply5/2, Delay4/1
  Multiply5/1 -> Add2/1
  Add2/1 -> Out_LoD_o/1
  Multiply4/1 -> Delay6/1
  Multiply3/1 -> Add3/1
  Delay4/1 -> Rate Transition/1
  LoD_1/1 -> Multiply5/1
  Delay6/1 -> Add3/2
  Rate Transition/1 -> Multiply3/2, Delay5/1

== system final_heart_sym3_3_Level_fixed/DWT_sym3_3_Level/1st_Level_Decomp1/HiD_Even ==
  In_HiD_e : Inport  OutDataTypeStr=fixdt(1,16,23)  SampleTime=1/44100
  Add : Sum  AccumDataTypeStr=fixdt(1,16,24)  OutDataTypeStr=fixdt(1,16,24)
  Add1 : Sum  AccumDataTypeStr=fixdt(1,16,24)  OutDataTypeStr=fixdt(1,16,25)
  Delay{,1..3} (4 alike) : Delay  DelayLength=1  SampleTime=1/44100
  HiD_0 : Constant  Value=-0.332670553  OutDataTypeStr=fixdt(1,16,16)  SampleTime=1/44100
  HiD_2 : Constant  Value=-0.459877502  OutDataTypeStr=fixdt(1,16,16)  SampleTime=1/44100
  HiD_4 : Constant  Value=0.085441274  OutDataTypeStr=fixdt(0,16,19)  SampleTime=1/44100
  Multiply1 : Product  OutDataTypeStr=fixdt(1,16,15)
  Multiply2 : Product  OutDataTypeStr=fixdt(0,16,28)
  Multiply3 : Product  OutDataTypeStr=fixdt(1,16,15)
  Rate Transition : RateTransition
  Rate Transition1 : RateTransition
  Out_HiD_e : Outport  OutDataTypeStr=fixdt(1,16,24)  SampleTime=1/44100  VectorParamsAs1DForOutWhenUnconnected=off
  wires:
  In_HiD_e/1 -> Multiply3/2, Delay/1
  Multiply3/1 -> Add/1
  HiD_0/1 -> Multiply3/1
  HiD_2/1 -> Multiply1/1
  Add/1 -> Out_HiD_e/1
  Multiply2/1 -> Delay2/1
  Multiply1/1 -> Add1/1
  Delay2/1 -> Add1/2
  Add1/1 -> Delay3/1
  Delay3/1 -> Add/2
  HiD_4/1 -> Multiply2/1
  Rate Transition1/1 -> Multiply2/2
  Delay1/1 -> Rate Transition1/1
  Rate Transition/1 -> Multiply1/2, Delay1/1
  Delay/1 -> Rate Transition/1

== system final_heart_sym3_3_Level_fixed/DWT_sym3_3_Level/1st_Level_Decomp1/HiD_Odd ==
  In_HiD_o : Inport  OutDataTypeStr=fixdt(1,16,23)  SampleTime=1/44100
  Add2 : Sum  AccumDataTypeStr=fixdt(1,16,23)  OutDataTypeStr=fixdt(1,16,24)
  Add3 : Sum  AccumDataTypeStr=fixdt(1,16,26)  OutDataTypeStr=fixdt(1,16,26)
  Delay{4..7} (4 alike) : Delay  DelayLength=1  SampleTime=1/44100
  HiD_1 : Constant  Value=0.806891509  OutDataTypeStr=fixdt(0,16,16)  SampleTime=1/44100
  HiD_3 : Constant  Value=-0.13501102  OutDataTypeStr=fixdt(1,16,17)  SampleTime=1/44100
  HiD_5 : Constant  Value=0.035226292  OutDataTypeStr=fixdt(0,16,20)  SampleTime=1/44100
  Multiply3 : Product  OutDataTypeStr=fixdt(1,16,15)
  Multiply4 : Product  OutDataTypeStr=fixdt(0,16,29)
  Multiply5 : Product  OutDataTypeStr=fixdt(0,16,24)
  Rate Transition : RateTransition
  Rate Transition1 : RateTransition
  Out_HiD_o : Outport  OutDataTypeStr=fixdt(1,16,24)  SampleTime=1/44100  VectorParamsAs1DForOutWhenUnconnected=off
  wires:
  Delay5/1 -> Rate Transition1/1
  Rate Transition1/1 -> Multiply4/2
  HiD_3/1 -> Multiply3/1
  Add3/1 -> Delay7/1
  Delay7/1 -> Add2/2
  HiD_5/1 -> Multiply4/1
  In_HiD_o/1 -> Multiply5/2, Delay4/1
  Multiply5/1 -> Add2/1
  Add2/1 -> Out_HiD_o/1
  Multiply4/1 -> Delay6/1
  Multiply3/1 -> Add3/1
  Delay4/1 -> Rate Transition/1
  HiD_1/1 -> Multiply5/1
  Delay6/1 -> Add3/2
  Rate Transition/1 -> Multiply3/2, Delay5/1

== system final_heart_sym3_3_Level_fixed/DWT_sym3_3_Level/1st_Level_Decomp1/LoD_Even ==
  In_LoD_e : Inport  OutDataTypeStr=fixdt(1,16,23)  SampleTime=1/44100
  Add2 : Sum  AccumDataTypeStr=fixdt(1,16,24)  OutDataTypeStr=fixdt(1,16,24)
  Add3 : Sum  AccumDataTypeStr=fixdt(1,16,23)  OutDataTypeStr=fixdt(1,16,24)
  Delay{4..7} (4 alike) : Delay  DelayLength=1  SampleTime=1/44100
  LoD_1 : Constant  Value=0.035226292  OutDataTypeStr=fixdt(0,16,20)  SampleTime=1/44100
  LoD_3 : Constant  Value=-0.13501102  OutDataTypeStr=fixdt(1,16,17)  SampleTime=1/44100
  LoD_5 : Constant  Value=0.806891509  OutDataTypeStr=fixdt(0,16,16)  SampleTime=1/44100
  Multiply3 : Product  OutDataTypeStr=fixdt(1,16,15)
  Multiply4 : Product  OutDataTypeStr=fixdt(0,16,24)
  Multiply5 : Product  OutDataTypeStr=fixdt(0,16,29)
  Rate Transition : RateTransition
  Rate Transition1 : RateTransition
  Out_LoD_e : Outport  OutDataTypeStr=fixdt(1,16,24)  SampleTime=1/44100  VectorParamsAs1DForOutWhenUnconnected=off
  wires:
  Delay5/1 -> Rate Transition1/1
  Rate Transition1/1 -> Multiply4/2
  LoD_3/1 -> Multiply3/1
  Add3/1 -> Delay7/1
  Delay7/1 -> Add2/2
  LoD_5/1 -> Multiply4/1
  In_LoD_e/1 -> Multiply5/2, Delay4/1
  Multiply5/1 -> Add2/1
  Add2/1 -> Out_LoD_e/1
  Multiply4/1 -> Delay6/1
  Multiply3/1 -> Add3/1
  Delay4/1 -> Rate Transition/1
  LoD_1/1 -> Multiply5/1
  Delay6/1 -> Add3/2
  Rate Transition/1 -> Multiply3/2, Delay5/1

== system final_heart_sym3_3_Level_fixed/DWT_sym3_3_Level/1st_Level_Decomp1/LoD_Odd ==
  In_LoD_o : Inport  OutDataTypeStr=fixdt(1,16,23)  SampleTime=1/44100
  Add2 : Sum  AccumDataTypeStr=fixdt(1,16,23)  OutDataTypeStr=fixdt(1,16,24)
  Add3 : Sum  AccumDataTypeStr=fixdt(0,16,24)  OutDataTypeStr=fixdt(0,16,24)
  Delay{4..7} (4 alike) : Delay  DelayLength=1  SampleTime=1/44100
  LoD_1 : Constant  Value=-0.085441274  OutDataTypeStr=fixdt(1,16,18)  SampleTime=1/44100
  LoD_3 : Constant  Value=0.459877502  OutDataTypeStr=fixdt(0,16,17)  SampleTime=1/44100
  LoD_5 : Constant  Value=0.332670553  OutDataTypeStr=fixdt(0,16,17)  SampleTime=1/44100
  Multiply3 : Product  OutDataTypeStr=fixdt(0,16,25)
  Multiply4 : Product  OutDataTypeStr=fixdt(0,16,26)
  Multiply5 : Product  OutDataTypeStr=fixdt(1,16,15)
  Rate Transition : RateTransition
  Rate Transition1 : RateTransition
  Out_LoD_o : Outport  OutDataTypeStr=fixdt(1,16,24)  SampleTime=1/44100  VectorParamsAs1DForOutWhenUnconnected=off
  wires:
  Delay5/1 -> Rate Transition1/1
  Rate Transition1/1 -> Multiply4/2
  LoD_3/1 -> Multiply3/1
  Add3/1 -> Delay7/1
  Delay7/1 -> Add2/2
  LoD_5/1 -> Multiply4/1
  In_LoD_o/1 -> Multiply5/2, Delay4/1
  Multiply5/1 -> Add2/1
  Add2/1 -> Out_LoD_o/1
  Multiply4/1 -> Delay6/1
  Multiply3/1 -> Add3/1
  Delay4/1 -> Rate Transition/1
  LoD_1/1 -> Multiply5/1
  Delay6/1 -> Add3/2
  Rate Transition/1 -> Multiply3/2, Delay5/1

== system final_heart_sym3_3_Level_fixed/DWT_sym3_3_Level/1st_Level_Decomp2/HiD_Even ==
  In_HiD_e : Inport  OutDataTypeStr=fixdt(1,16,24)  SampleTime=1/44100
  Add : Sum  AccumDataTypeStr=fixdt(1,16,24)  OutDataTypeStr=fixdt(1,16,24)
  Add1 : Sum  AccumDataTypeStr=fixdt(1,16,25)  OutDataTypeStr=fixdt(1,16,25)
  Delay{,1..3} (4 alike) : Delay  DelayLength=1  SampleTime=1/44100
  HiD_0 : Constant  Value=-0.332670553  OutDataTypeStr=fixdt(1,16,16)  SampleTime=1/44100
  HiD_2 : Constant  Value=-0.459877502  OutDataTypeStr=fixdt(1,16,16)  SampleTime=1/44100
  HiD_4 : Constant  Value=0.085441274  OutDataTypeStr=fixdt(0,16,19)  SampleTime=1/44100
  Multiply1 : Product  OutDataTypeStr=fixdt(1,16,15)
  Multiply2 : Product  OutDataTypeStr=fixdt(0,16,28)
  Multiply3 : Product  OutDataTypeStr=fixdt(1,16,15)
  Rate Transition : RateTransition
  Rate Transition1 : RateTransition
  Out_HiD_e : Outport  OutDataTypeStr=fixdt(1,16,24)  SampleTime=1/44100  VectorParamsAs1DForOutWhenUnconnected=off
  wires:
  In_HiD_e/1 -> Multiply3/2, Delay/1
  Multiply3/1 -> Add/1
  HiD_0/1 -> Multiply3/1
  HiD_2/1 -> Multiply1/1
  Add/1 -> Out_HiD_e/1
  Multiply2/1 -> Delay2/1
  Multiply1/1 -> Add1/1
  Delay2/1 -> Add1/2
  Add1/1 -> Delay3/1
  Delay3/1 -> Add/2
  HiD_4/1 -> Multiply2/1
  Rate Transition1/1 -> Multiply2/2
  Delay1/1 -> Rate Transition1/1
  Rate Transition/1 -> Multiply1/2, Delay1/1
  Delay/1 -> Rate Transition/1

== system final_heart_sym3_3_Level_fixed/DWT_sym3_3_Level/1st_Level_Decomp2/HiD_Odd ==
  In_HiD_o : Inport  OutDataTypeStr=fixdt(1,16,24)  SampleTime=1/44100
  Add2 : Sum  AccumDataTypeStr=fixdt(1,16,24)  OutDataTypeStr=fixdt(1,16,24)
  Add3 : Sum  AccumDataTypeStr=fixdt(1,16,26)  OutDataTypeStr=fixdt(1,16,27)
  Delay{4..7} (4 alike) : Delay  DelayLength=1  SampleTime=1/44100
  HiD_1 : Constant  Value=0.806891509  OutDataTypeStr=fixdt(0,16,16)  SampleTime=1/44100
  HiD_3 : Constant  Value=-0.13501102  OutDataTypeStr=fixdt(1,16,17)  SampleTime=1/44100
  HiD_5 : Constant  Value=0.035226292  OutDataTypeStr=fixdt(0,16,20)  SampleTime=1/44100
  Multiply3 : Product  OutDataTypeStr=fixdt(1,16,15)
  Multiply4 : Product  OutDataTypeStr=fixdt(0,16,29)
  Multiply5 : Product  OutDataTypeStr=fixdt(0,16,25)
  Rate Transition : RateTransition
  Rate Transition1 : RateTransition
  Out_HiD_o : Outport  OutDataTypeStr=fixdt(1,16,24)  SampleTime=1/44100  VectorParamsAs1DForOutWhenUnconnected=off
  wires:
  Delay5/1 -> Rate Transition1/1
  Rate Transition1/1 -> Multiply4/2
  HiD_3/1 -> Multiply3/1
  Add3/1 -> Delay7/1
  Delay7/1 -> Add2/2
  HiD_5/1 -> Multiply4/1
  In_HiD_o/1 -> Multiply5/2, Delay4/1
  Multiply5/1 -> Add2/1
  Add2/1 -> Out_HiD_o/1
  Multiply4/1 -> Delay6/1
  Multiply3/1 -> Add3/1
  Delay4/1 -> Rate Transition/1
  HiD_1/1 -> Multiply5/1
  Delay6/1 -> Add3/2
  Rate Transition/1 -> Multiply3/2, Delay5/1

== system final_heart_sym3_3_Level_fixed/DWT_sym3_3_Level/1st_Level_Decomp2/LoD_Even ==
  In_LoD_e : Inport  OutDataTypeStr=fixdt(1,16,24)  SampleTime=1/44100
  Add2 : Sum  AccumDataTypeStr=fixdt(1,16,24)  OutDataTypeStr=fixdt(1,16,24)
  Add3 : Sum  AccumDataTypeStr=fixdt(1,16,24)  OutDataTypeStr=fixdt(1,16,24)
  Delay{4..7} (4 alike) : Delay  DelayLength=1  SampleTime=1/44100
  LoD_1 : Constant  Value=0.035226292  OutDataTypeStr=fixdt(0,16,20)  SampleTime=1/44100
  LoD_3 : Constant  Value=-0.13501102  OutDataTypeStr=fixdt(1,16,17)  SampleTime=1/44100
  LoD_5 : Constant  Value=0.806891509  OutDataTypeStr=fixdt(0,16,16)  SampleTime=1/44100
  Multiply3 : Product  OutDataTypeStr=fixdt(1,16,15)
  Multiply4 : Product  OutDataTypeStr=fixdt(0,16,25)
  Multiply5 : Product  OutDataTypeStr=fixdt(0,16,29)
  Rate Transition : RateTransition
  Rate Transition1 : RateTransition
  Out_LoD_e : Outport  OutDataTypeStr=fixdt(1,16,24)  SampleTime=1/44100  VectorParamsAs1DForOutWhenUnconnected=off
  wires:
  Delay5/1 -> Rate Transition1/1
  Rate Transition1/1 -> Multiply4/2
  LoD_3/1 -> Multiply3/1
  Add3/1 -> Delay7/1
  Delay7/1 -> Add2/2
  LoD_5/1 -> Multiply4/1
  In_LoD_e/1 -> Multiply5/2, Delay4/1
  Multiply5/1 -> Add2/1
  Add2/1 -> Out_LoD_e/1
  Multiply4/1 -> Delay6/1
  Multiply3/1 -> Add3/1
  Delay4/1 -> Rate Transition/1
  LoD_1/1 -> Multiply5/1
  Delay6/1 -> Add3/2
  Rate Transition/1 -> Multiply3/2, Delay5/1

== system final_heart_sym3_3_Level_fixed/DWT_sym3_3_Level/1st_Level_Decomp2/LoD_Odd ==
  In_LoD_o : Inport  OutDataTypeStr=fixdt(1,16,24)  SampleTime=1/44100
  Add2 : Sum  AccumDataTypeStr=fixdt(1,16,24)  OutDataTypeStr=fixdt(1,16,24)
  Add3 : Sum  AccumDataTypeStr=fixdt(0,16,25)  OutDataTypeStr=fixdt(0,16,25)
  Delay{4..7} (4 alike) : Delay  DelayLength=1  SampleTime=1/44100
  LoD_1 : Constant  Value=-0.085441274  OutDataTypeStr=fixdt(1,16,18)  SampleTime=1/44100
  LoD_3 : Constant  Value=0.459877502  OutDataTypeStr=fixdt(0,16,17)  SampleTime=1/44100
  LoD_5 : Constant  Value=0.332670553  OutDataTypeStr=fixdt(0,16,17)  SampleTime=1/44100
  Multiply3 : Product  OutDataTypeStr=fixdt(0,16,26)
  Multiply4 : Product  OutDataTypeStr=fixdt(0,16,26)
  Multiply5 : Product  OutDataTypeStr=fixdt(1,16,15)
  Rate Transition : RateTransition
  Rate Transition1 : RateTransition
  Out_LoD_o : Outport  OutDataTypeStr=fixdt(1,16,24)  SampleTime=1/44100  VectorParamsAs1DForOutWhenUnconnected=off
  wires:
  Delay5/1 -> Rate Transition1/1
  Rate Transition1/1 -> Multiply4/2
  LoD_3/1 -> Multiply3/1
  Add3/1 -> Delay7/1
  Delay7/1 -> Add2/2
  LoD_5/1 -> Multiply4/1
  In_LoD_o/1 -> Multiply5/2, Delay4/1
  Multiply5/1 -> Add2/1
  Add2/1 -> Out_LoD_o/1
  Multiply4/1 -> Delay6/1
  Multiply3/1 -> Add3/1
  Delay4/1 -> Rate Transition/1
  LoD_1/1 -> Multiply5/1
  Delay6/1 -> Add3/2
  Rate Transition/1 -> Multiply3/2, Delay5/1

== system final_heart_sym3_3_Level_fixed/DWT_sym3_3_Level/1st_Level_Recon/HiR_Even ==
  In_HiR_e : Inport  OutDataTypeStr=fixdt(1,16,28)  SampleTime=1/44100
  Add : Sum  AccumDataTypeStr=fixdt(1,16,28)  OutDataTypeStr=fixdt(1,16,28)
  Add1 : Sum  AccumDataTypeStr=fixdt(1,16,28)  OutDataTypeStr=fixdt(1,16,28)
  Delay{,1..3} (4 alike) : Delay  DelayLength=1  SampleTime=1/44100
  HiR_0 : Constant  Value=0.035226292  OutDataTypeStr=fixdt(0,16,20)  SampleTime=1/44100
  HiR_2 : Constant  Value=-0.13501102  OutDataTypeStr=fixdt(1,16,17)  SampleTime=1/44100
  HiR_4 : Constant  Value=0.806891509  OutDataTypeStr=fixdt(0,16,16)  SampleTime=1/44100
  Multiply : Product  OutDataTypeStr=fixdt(1,16,33)
  Multiply1 : Product  OutDataTypeStr=fixdt(1,16,31)
  Multiply2 : Product  OutDataTypeStr=fixdt(1,16,28)
  Rate Transition : RateTransition
  Rate Transition1 : RateTransition
  Out_HiR_e : Outport  OutDataTypeStr=fixdt(1,16,28)  SampleTime=1/44100  VectorParamsAs1DForOutWhenUnconnected=off
  wires:
  Delay3/1 -> Add/2
  In_HiR_e/1 -> Delay/1, Multiply/2
  HiR_4/1 -> Multiply2/1
  Multiply/1 -> Add/1
  Add1/1 -> Delay3/1
  Multiply2/1 -> Delay2/1
  Multiply1/1 -> Add1/1
  Delay2/1 -> Add1/2
  Add/1 -> Out_HiR_e/1
  HiR_0/1 -> Multiply/1
  HiR_2/1 -> Multiply1/1
  Delay1/1 -> Rate Transition1/1
  Rate Transition/1 -> Delay1/1, Multiply1/2
  Rate Transition1/1 -> Multiply2/2
  Delay/1 -> Rate Transition/1

== system final_heart_sym3_3_Level_fixed/DWT_sym3_3_Level/1st_Level_Recon/HiR_Odd ==
  In_HiR_o : Inport  OutDataTypeStr=fixdt(1,16,28)  SampleTime=1/44100
  Add : Sum  AccumDataTypeStr=fixdt(1,16,29)  OutDataTypeStr=fixdt(1,16,29)
  Add1 : Sum  AccumDataTypeStr=fixdt(1,16,29)  OutDataTypeStr=fixdt(1,16,29)
  Delay{,1..3} (4 alike) : Delay  DelayLength=1  SampleTime=1/44100
  HiR_1 : Constant  Value=0.085441274  OutDataTypeStr=fixdt(0,16,19)  SampleTime=1/44100
  HiR_3 : Constant  Value=-0.459877502  OutDataTypeStr=fixdt(1,16,16)  SampleTime=1/44100
  HiR_5 : Constant  Value=-0.332670553  OutDataTypeStr=fixdt(1,16,16)  SampleTime=1/44100
  Multiply : Product  OutDataTypeStr=fixdt(1,16,31)
  Multiply1 : Product  OutDataTypeStr=fixdt(1,16,29)
  Multiply2 : Product  OutDataTypeStr=fixdt(1,16,30)
  Rate Transition : RateTransition
  Rate Transition1 : RateTransition
  Out_HiR_o : Outport  OutDataTypeStr=fixdt(1,16,29)  SampleTime=1/44100  VectorParamsAs1DForOutWhenUnconnected=off
  wires:
  Delay/1 -> Rate Transition/1
  Rate Transition1/1 -> Multiply2/2
  Delay2/1 -> Add1/2
  HiR_1/1 -> Multiply/1
  Add/1 -> Out_HiR_o/1
  Delay1/1 -> Rate Transition1/1
  HiR_3/1 -> Multiply1/1
  Multiply1/1 -> Add1/1
  Rate Transition/1 -> Delay1/1, Multiply1/2
  Add1/1 -> Delay3/1
  Multiply/1 -> Add/1
  In_HiR_o/1 -> Delay/1, Multiply/2
  Multiply2/1 -> Delay2/1
  HiR_5/1 -> Multiply2/1
  Delay3/1 -> Add/2

== system final_heart_sym3_3_Level_fixed/DWT_sym3_3_Level/1st_Level_Recon/LoR_Even ==
  In_LoR_e : Inport  OutDataTypeStr=fixdt(1,16,24)  SampleTime=1/44100
  Add : Sum  AccumDataTypeStr=fixdt(1,16,24)  OutDataTypeStr=fixdt(1,16,24)
  Add1 : Sum  AccumDataTypeStr=fixdt(1,16,25)  OutDataTypeStr=fixdt(1,16,25)
  Delay{,1..3} (4 alike) : Delay  DelayLength=1  SampleTime=1/44100
  LoR_0 : Constant  Value=0.332670553  OutDataTypeStr=fixdt(0,16,17)  SampleTime=1/44100
  LoR_2 : Constant  Value=0.459877502  OutDataTypeStr=fixdt(0,16,17)  SampleTime=1/44100
  LoR_4 : Constant  Value=-0.085441274  OutDataTypeStr=fixdt(1,16,18)  SampleTime=1/44100
  Multiply : Product  OutDataTypeStr=fixdt(1,16,26)
  Multiply1 : Product  OutDataTypeStr=fixdt(1,16,25)
  Multiply2 : Product  OutDataTypeStr=fixdt(1,16,27)
  Rate Transition : RateTransition
  Rate Transition1 : RateTransition
  Out_LoR_e : Outport  OutDataTypeStr=fixdt(1,16,24)  SampleTime=1/44100  VectorParamsAs1DForOutWhenUnconnected=off
  wires:
  Delay/1 -> Rate Transition/1
  Rate Transition1/1 -> Multiply2/2
  Delay2/1 -> Add1/2
  LoR_0/1 -> Multiply/1
  Add/1 -> Out_LoR_e/1
  Delay1/1 -> Rate Transition1/1
  LoR_2/1 -> Multiply1/1
  Multiply1/1 -> Add1/1
  Rate Transition/1 -> Delay1/1, Multiply1/2
  Add1/1 -> Delay3/1
  Multiply/1 -> Add/1
  In_LoR_e/1 -> Delay/1, Multiply/2
  Multiply2/1 -> Delay2/1
  LoR_4/1 -> Multiply2/1
  Delay3/1 -> Add/2

== system final_heart_sym3_3_Level_fixed/DWT_sym3_3_Level/1st_Level_Recon/LoR_Odd ==
  In_LoR_o : Inport  OutDataTypeStr=fixdt(1,16,24)  SampleTime=1/44100
  Add : Sum  AccumDataTypeStr=fixdt(1,16,24)  OutDataTypeStr=fixdt(1,16,24)
  Add1 : Sum  AccumDataTypeStr=fixdt(1,16,27)  OutDataTypeStr=fixdt(1,16,27)
  Delay{,1..3} (4 alike) : Delay  DelayLength=1  SampleTime=1/44100
  LoR_1 : Constant  Value=0.806891509  OutDataTypeStr=fixdt(0,16,16)  SampleTime=1/44100
  LoR_3 : Constant  Value=-0.13501102  OutDataTypeStr=fixdt(1,16,17)  SampleTime=1/44100
  LoR_5 : Constant  Value=0.035226292  OutDataTypeStr=fixdt(0,16,20)  SampleTime=1/44100
  Multiply : Product  OutDataTypeStr=fixdt(1,16,24)
  Multiply1 : Product  OutDataTypeStr=fixdt(1,16,27)
  Multiply2 : Product  OutDataTypeStr=fixdt(1,16,29)
  Rate Transition : RateTransition
  Rate Transition1 : RateTransition
  Out_LoR_o : Outport  OutDataTypeStr=fixdt(1,16,24)  SampleTime=1/44100  VectorParamsAs1DForOutWhenUnconnected=off
  wires:
  Delay/1 -> Rate Transition/1
  Rate Transition1/1 -> Multiply2/2
  Delay2/1 -> Add1/2
  LoR_1/1 -> Multiply/1
  Add/1 -> Out_LoR_o/1
  Delay1/1 -> Rate Transition1/1
  LoR_3/1 -> Multiply1/1
  Multiply1/1 -> Add1/1
  Rate Transition/1 -> Delay1/1, Multiply1/2
  Add1/1 -> Delay3/1
  Multiply/1 -> Add/1
  In_LoR_o/1 -> Delay/1, Multiply/2
  Multiply2/1 -> Delay2/1
  LoR_5/1 -> Multiply2/1
  Delay3/1 -> Add/2

== system final_heart_sym3_3_Level_fixed/DWT_sym3_3_Level/1st_Level_Recon1/HiR_Even ==
  In_HiR_e : Inport  OutDataTypeStr=fixdt(1,16,28)  SampleTime=1/44100
  Add : Sum  AccumDataTypeStr=fixdt(1,16,28)  OutDataTypeStr=fixdt(1,16,28)
  Add1 : Sum  AccumDataTypeStr=fixdt(1,16,28)  OutDataTypeStr=fixdt(1,16,28)
  Delay{,1..3} (4 alike) : Delay  DelayLength=1  SampleTime=1/44100
  HiR_0 : Constant  Value=0.035226292  OutDataTypeStr=fixdt(0,16,20)  SampleTime=1/44100
  HiR_2 : Constant  Value=-0.13501102  OutDataTypeStr=fixdt(1,16,17)  SampleTime=1/44100
  HiR_4 : Constant  Value=0.806891509  OutDataTypeStr=fixdt(0,16,16)  SampleTime=1/44100
  Multiply : Product  OutDataTypeStr=fixdt(1,16,33)
  Multiply1 : Product  OutDataTypeStr=fixdt(1,16,31)
  Multiply2 : Product  OutDataTypeStr=fixdt(1,16,28)
  Rate Transition : RateTransition
  Rate Transition1 : RateTransition
  Out_HiR_e : Outport  OutDataTypeStr=fixdt(1,16,28)  SampleTime=1/44100  VectorParamsAs1DForOutWhenUnconnected=off
  wires:
  Delay3/1 -> Add/2
  In_HiR_e/1 -> Delay/1, Multiply/2
  HiR_4/1 -> Multiply2/1
  Multiply/1 -> Add/1
  Add1/1 -> Delay3/1
  Multiply2/1 -> Delay2/1
  Multiply1/1 -> Add1/1
  Delay2/1 -> Add1/2
  Add/1 -> Out_HiR_e/1
  HiR_0/1 -> Multiply/1
  HiR_2/1 -> Multiply1/1
  Delay1/1 -> Rate Transition1/1
  Rate Transition/1 -> Delay1/1, Multiply1/2
  Rate Transition1/1 -> Multiply2/2
  Delay/1 -> Rate Transition/1

== system final_heart_sym3_3_Level_fixed/DWT_sym3_3_Level/1st_Level_Recon1/HiR_Odd ==
  In_HiR_o : Inport  OutDataTypeStr=fixdt(1,16,28)  SampleTime=1/44100
  Add : Sum  AccumDataTypeStr=fixdt(1,16,29)  OutDataTypeStr=fixdt(1,16,29)
  Add1 : Sum  AccumDataTypeStr=fixdt(1,16,29)  OutDataTypeStr=fixdt(1,16,29)
  Delay{,1..3} (4 alike) : Delay  DelayLength=1  SampleTime=1/44100
  HiR_1 : Constant  Value=0.085441274  OutDataTypeStr=fixdt(0,16,19)  SampleTime=1/44100
  HiR_3 : Constant  Value=-0.459877502  OutDataTypeStr=fixdt(1,16,16)  SampleTime=1/44100
  HiR_5 : Constant  Value=-0.332670553  OutDataTypeStr=fixdt(1,16,16)  SampleTime=1/44100
  Multiply : Product  OutDataTypeStr=fixdt(1,16,31)
  Multiply1 : Product  OutDataTypeStr=fixdt(1,16,29)
  Multiply2 : Product  OutDataTypeStr=fixdt(1,16,30)
  Rate Transition : RateTransition
  Rate Transition1 : RateTransition
  Out_HiR_o : Outport  OutDataTypeStr=fixdt(1,16,29)  SampleTime=1/44100  VectorParamsAs1DForOutWhenUnconnected=off
  wires:
  Delay/1 -> Rate Transition/1
  Rate Transition1/1 -> Multiply2/2
  Delay2/1 -> Add1/2
  HiR_1/1 -> Multiply/1
  Add/1 -> Out_HiR_o/1
  Delay1/1 -> Rate Transition1/1
  HiR_3/1 -> Multiply1/1
  Multiply1/1 -> Add1/1
  Rate Transition/1 -> Delay1/1, Multiply1/2
  Add1/1 -> Delay3/1
  Multiply/1 -> Add/1
  In_HiR_o/1 -> Delay/1, Multiply/2
  Multiply2/1 -> Delay2/1
  HiR_5/1 -> Multiply2/1
  Delay3/1 -> Add/2

== system final_heart_sym3_3_Level_fixed/DWT_sym3_3_Level/1st_Level_Recon1/LoR_Even ==
  In_LoR_e : Inport  OutDataTypeStr=fixdt(1,16,24)  SampleTime=1/44100
  Add : Sum  AccumDataTypeStr=fixdt(1,16,24)  OutDataTypeStr=fixdt(1,16,24)
  Add1 : Sum  AccumDataTypeStr=fixdt(1,16,25)  OutDataTypeStr=fixdt(1,16,25)
  Delay{,1..3} (4 alike) : Delay  DelayLength=1  SampleTime=1/44100
  LoR_0 : Constant  Value=0.332670553  OutDataTypeStr=fixdt(0,16,17)  SampleTime=1/44100
  LoR_2 : Constant  Value=0.459877502  OutDataTypeStr=fixdt(0,16,17)  SampleTime=1/44100
  LoR_4 : Constant  Value=-0.085441274  OutDataTypeStr=fixdt(1,16,18)  SampleTime=1/44100
  Multiply : Product  OutDataTypeStr=fixdt(1,16,25)
  Multiply1 : Product  OutDataTypeStr=fixdt(1,16,25)
  Multiply2 : Product  OutDataTypeStr=fixdt(1,16,27)
  Rate Transition : RateTransition
  Rate Transition1 : RateTransition
  Out_LoR_e : Outport  OutDataTypeStr=fixdt(1,16,24)  SampleTime=1/44100  VectorParamsAs1DForOutWhenUnconnected=off
  wires:
  Delay/1 -> Rate Transition/1
  Rate Transition1/1 -> Multiply2/2
  Delay2/1 -> Add1/2
  LoR_0/1 -> Multiply/1
  Add/1 -> Out_LoR_e/1
  Delay1/1 -> Rate Transition1/1
  LoR_2/1 -> Multiply1/1
  Multiply1/1 -> Add1/1
  Rate Transition/1 -> Delay1/1, Multiply1/2
  Add1/1 -> Delay3/1
  Multiply/1 -> Add/1
  In_LoR_e/1 -> Delay/1, Multiply/2
  Multiply2/1 -> Delay2/1
  LoR_4/1 -> Multiply2/1
  Delay3/1 -> Add/2

== system final_heart_sym3_3_Level_fixed/DWT_sym3_3_Level/1st_Level_Recon1/LoR_Odd ==
  In_LoR_o : Inport  OutDataTypeStr=fixdt(1,16,24)  SampleTime=1/44100
  Add : Sum  AccumDataTypeStr=fixdt(1,16,24)  OutDataTypeStr=fixdt(1,16,24)
  Add1 : Sum  AccumDataTypeStr=fixdt(1,16,26)  OutDataTypeStr=fixdt(1,16,27)
  Delay{,1..3} (4 alike) : Delay  DelayLength=1  SampleTime=1/44100
  LoR_1 : Constant  Value=0.806891509  OutDataTypeStr=fixdt(0,16,16)  SampleTime=1/44100
  LoR_3 : Constant  Value=-0.13501102  OutDataTypeStr=fixdt(1,16,17)  SampleTime=1/44100
  LoR_5 : Constant  Value=0.035226292  OutDataTypeStr=fixdt(0,16,20)  SampleTime=1/44100
  Multiply : Product  OutDataTypeStr=fixdt(1,16,24)
  Multiply1 : Product  OutDataTypeStr=fixdt(1,16,26)
  Multiply2 : Product  OutDataTypeStr=fixdt(1,16,28)
  Rate Transition : RateTransition
  Rate Transition1 : RateTransition
  Out_LoR_o : Outport  OutDataTypeStr=fixdt(1,16,24)  SampleTime=1/44100  VectorParamsAs1DForOutWhenUnconnected=off
  wires:
  Delay/1 -> Rate Transition/1
  Rate Transition1/1 -> Multiply2/2
  Delay2/1 -> Add1/2
  LoR_1/1 -> Multiply/1
  Add/1 -> Out_LoR_o/1
  Delay1/1 -> Rate Transition1/1
  LoR_3/1 -> Multiply1/1
  Multiply1/1 -> Add1/1
  Rate Transition/1 -> Delay1/1, Multiply1/2
  Add1/1 -> Delay3/1
  Multiply/1 -> Add/1
  In_LoR_o/1 -> Delay/1, Multiply/2
  Multiply2/1 -> Delay2/1
  LoR_5/1 -> Multiply2/1
  Delay3/1 -> Add/2
